simulink model "ATV7_2_SIMULINK"  (R2021a)
settings: Solver=VariableStepAuto  StartTime=0.0  StopTime=1.5  RelTol=1e-3
settings Model: Creator=Home  LastModifiedBy=Home

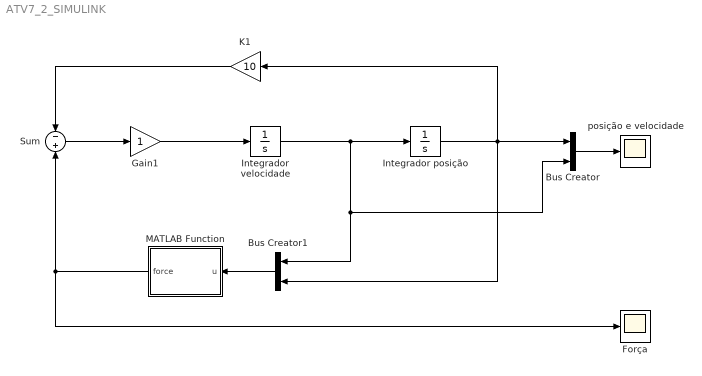
== system ATV7_2_SIMULINK ==
  Bus Creator : BusCreator  Inputs=2
  Bus Creator1 : BusCreator  Inputs=2
  Força : Scope
  Gain1 : Gain
  Integrador posição : Integrator  InitialCondition=0.05
  Integrador velocidade : Integrator  InitialCondition=-0.5
  K1 : Gain  Gain=10
  MATLAB Function : MATLAB Function  TreatAsAtomicUnit=on
  Sum : Sum  Inputs=-|+
  posição e velocidade : Scope
  wires:
  Sum/1 -> Gain1/1
  Bus Creator/1 -> posição e velocidade/1
  Integrador velocidade/1 -> Integrador posição/1, Bus Creator/2, Bus Creator1/1
  K1/1 -> Sum/1
  Gain1/1 -> Integrador velocidade/1
  MATLAB Function/1(force) -> Força/1, Sum/2
  Bus Creator1/1 -> MATLAB Function/1(u)
  Integrador posição/1 -> K1/1, Bus Creator1/2, Bus Creator/1

== matlab function ATV7_2_SIMULINK/MATLAB Function ==
  data: u input; force output
function force = fsnub(u)
    % FSNUB computes the nonlinear force for snubber simulation
    %
    % Computes the snubber force as a function of
    % displacement and velocity
    %
    % u(1) = displacement ; x(0) = 0.05 != -0.5 => portante esta variavel
    %                                              é a velocidade
    % u(2) = velocity

    xsnub = -0.05; % Location of snubber
    k2 = 50.0; % Spring constant (N/m)
    b = 50.0; % Damping (Ns/m)

    disp(u(1));
    
    if u(2) > xsnub
        force = 0.0; % not in contact
    else
        force = k2*(xsnub - u(2)) - b*u(1);
    end

    % Snubber cannot exert a negative force
    if force < 0
        force = 0;
    end
